simulink model "lowConnectivity"  (Simulink 9.3)
settings: Solver=ode4  StartTime=0.0  StopTime=60  FixedStep=.004  RelTol=1e-3  EnableMultiTasking=on
Description:
  | Author: Ali Najmaldin
settings Model: Creator=Author: Ali Najmaldin  LastModifiedBy=alinajmaldin  SimulationMode=accelerator
settings DataIOCC: SaveOutput=off  SignalLogging=off  SaveTime=off
settings OptimizationCC: ExpressionDepthLimit=2147483647
settings DebuggingCC: SaveWithParameterizedLinksMsg=none  SolverPrmCheckMsg=warning  InheritedTsInSrcMsg=none  ModelReferenceDataLoggingMessage=none  StateNameClashWarn=warning
settings SFSimCC: SimParseCustomCode=off

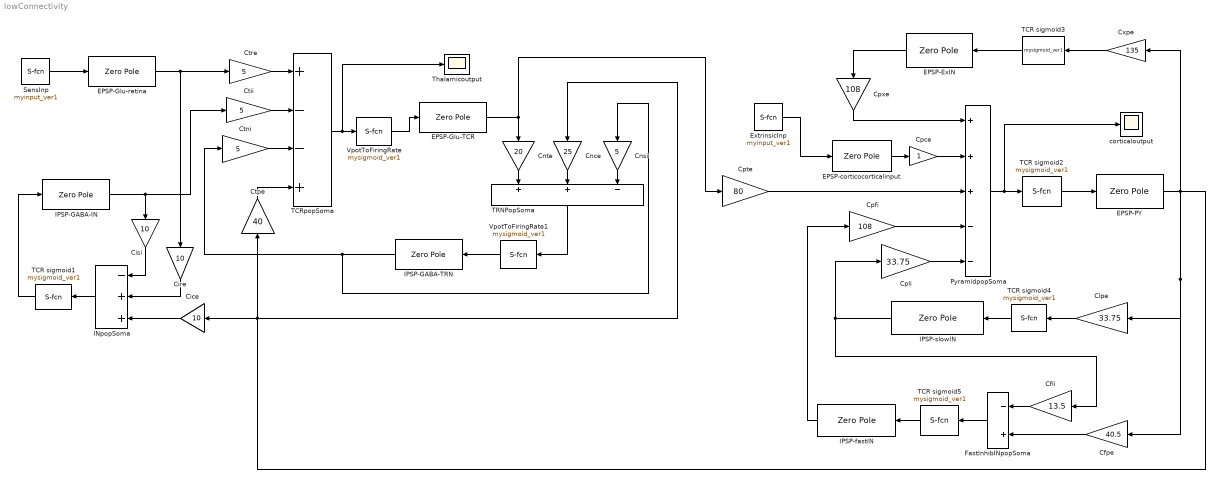
== system lowConnectivity ==
  Cfli : Gain  Gain=13.5
  Cfpe : Gain  Gain=40.5
  Cice : Gain  Gain=10
  Cire : Gain  Gain=10
  Cisi : Gain  Gain=10
  Clpe : Gain  Gain=33.75
  Cnce : Gain  Gain=25
  Cnsi : Gain  Gain=5
  Cnte : Gain  Gain=20
  Cpce : Gain
  Cpfi : Gain  Gain=108
  Cpli : Gain  Gain=33.75
  Cpte : Gain  Gain=80
  Cpxe : Gain  Gain=108
  Ctii : Gain  Gain=5
  Ctni : Gain  Gain=5
  Ctpe : Gain  Gain=40
  Ctre : Gain  Gain=5
  Cxpe : Gain  Gain=135
  EPSP-ExIN : ZeroPole  Zeros=[]  Poles=[-40 -40]  Gain=[40* 0.0027]
  EPSP-Glu-TCR : ZeroPole  Zeros=[]  Poles=[-100 -100]  Gain=[0.00325*100]
  EPSP-Glu-retina : ZeroPole  Zeros=[]  Poles=[-100 -100]  Gain=[0.00325*100]
  EPSP-PY : ZeroPole  Zeros=[]  Poles=[-40 -40]  Gain=[40* 0.0027]
  EPSP-corticocorticalinput : ZeroPole  Zeros=[]  Poles=[-40 -40]  Gain=[40* 0.0027]
  ExtrinsicInp : M-S-Function  Description=|  FunctionName=myinput_ver1  Parameters=30,5,60000,1
      | Input to the model with or without noise. The order of input parameters in the Dialog box is:                      
      | mean, standard deviation, length of signal,flag,constant.                                                          
      | If flag is 0, the input is a constant devoid of any noise. However, if flag is 1, the noise is added to the signal.
      mask Display: plot(312+randn(1,25))
  FastInhibINpopSoma : Sum  Inputs=-+  CollapseMode=Specified dimension  CollapseDim=4
  INpopSoma : Sum  Inputs=-++  CollapseMode=Specified dimension  CollapseDim=4
  IPSP-GABA-IN : ZeroPole  Zeros=[]  Poles=[-40 -40]  Gain=[0.022*40]
  IPSP-GABA-TRN : ZeroPole  Zeros=[]  Poles=[-40 -40]  Gain=[0.022*40]
  IPSP-fastIN : ZeroPole  Zeros=[]  Poles=[-300 -300]  Gain=[300*0.039]
  IPSP-slowIN : ZeroPole  Zeros=[]  Poles=[-20 -20]  Gain=[20*0.0045]
  PyramidpopSoma : Sum  Inputs=+++--  CollapseMode=Specified dimension  CollapseDim=4
  SensInp : M-S-Function  Description=|  FunctionName=myinput_ver1  Parameters=11,5,60000,1
      | Input to the model with or without noise. The order of input parameters in the Dialog box is:                      
      | mean, standard deviation, length of signal,flag,constant.                                                          
      | If flag is 0, the input is a constant devoid of any noise. However, if flag is 1, the noise is added to the signal.
      mask Display: plot(312+randn(1,25))
  TCR sigmoid{1..5} (5 alike) : M-S-Function  FunctionName=mysigmoid_ver1  Parameters=2.5,560,0.006
      mask Display: plot(1./(1+exp(-0.75.*([1:25]-12))))
  TCRpopSoma : Sum  Inputs=+--+  CollapseMode=Specified dimension  CollapseDim=4
  TRNPopSoma : Sum  Inputs=++-  CollapseMode=Specified dimension  CollapseDim=4
  Thalamicoutput : Scope
  VpotToFiringRate : M-S-Function  FunctionName=mysigmoid_ver1  Parameters=2.5,560,0.006
      mask Display: plot(1./(1+exp(-0.75.*([1:25]-12))))
  VpotToFiringRate1 : M-S-Function  FunctionName=mysigmoid_ver1  Parameters=2.5,560,0.006
      mask Display: plot(1./(1+exp(-0.75.*([1:25]-12))))
  corticaloutput : Scope
  wires:
  Ctre/1 -> TCRpopSoma/1
  SensInp/1 -> EPSP-Glu-retina/1
  EPSP-Glu-retina/1 -> Ctre/1, Cire/1
  TCRpopSoma/1 -> VpotToFiringRate/1, Thalamicoutput/1
  INpopSoma/1 -> TCR sigmoid1/1
  Cire/1 -> INpopSoma/2
  TCR sigmoid1/1 -> IPSP-GABA-IN/1
  IPSP-GABA-IN/1 -> Ctii/1, Cisi/1
  TRNPopSoma/1 -> VpotToFiringRate1/1
  VpotToFiringRate/1 -> EPSP-Glu-TCR/1
  Cnte/1 -> TRNPopSoma/1
  VpotToFiringRate1/1 -> IPSP-GABA-TRN/1
  IPSP-GABA-TRN/1 -> Ctni/1, Cnsi/1
  Cnce/1 -> TRNPopSoma/2
  Ctii/1 -> TCRpopSoma/2
  Ctni/1 -> TCRpopSoma/3
  Ctpe/1 -> TCRpopSoma/4
  Cisi/1 -> INpopSoma/1
  Cice/1 -> INpopSoma/3
  Cnsi/1 -> TRNPopSoma/3
  EPSP-Glu-TCR/1 -> Cnte/1, Cpte/1
  PyramidpopSoma/1 -> TCR sigmoid2/1, corticaloutput/1
  TCR sigmoid2/1 -> EPSP-PY/1
  Cxpe/1 -> TCR sigmoid3/1
  TCR sigmoid3/1 -> EPSP-ExIN/1
  Clpe/1 -> TCR sigmoid4/1
  TCR sigmoid4/1 -> IPSP-slowIN/1
  IPSP-slowIN/1 -> Cpli/1, Cfli/1
  Cfli/1 -> FastInhibINpopSoma/1
  TCR sigmoid5/1 -> IPSP-fastIN/1
  IPSP-fastIN/1 -> Cpfi/1
  EPSP-ExIN/1 -> Cpxe/1
  EPSP-PY/1 -> Clpe/1, Cfpe/1, Cxpe/1, Ctpe/1, Cice/1, Cnce/1
  FastInhibINpopSoma/1 -> TCR sigmoid5/1
  Cfpe/1 -> FastInhibINpopSoma/2
  ExtrinsicInp/1 -> EPSP-corticocorticalinput/1
  Cpxe/1 -> PyramidpopSoma/1
  EPSP-corticocorticalinput/1 -> Cpce/1
  Cpfi/1 -> PyramidpopSoma/4
  Cpli/1 -> PyramidpopSoma/5
  Cpte/1 -> PyramidpopSoma/3
  Cpce/1 -> PyramidpopSoma/2
